simulink library "momentum_dump_lib"  (R2016b)
settings: Solver=VariableStepAuto  StartTime=0.0  StopTime=10.0  RelTol=1e-3
undefined symbols (not defined in the file or in its folder): fsw_params
libraries: vrlib x1, dspmathops x1
settings Model: Creator=unsik  LastModifiedBy=Taylor

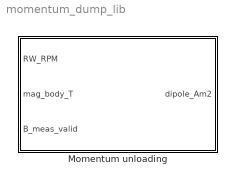
== system momentum_dump_lib ==
  Momentum unloading : Subsystem

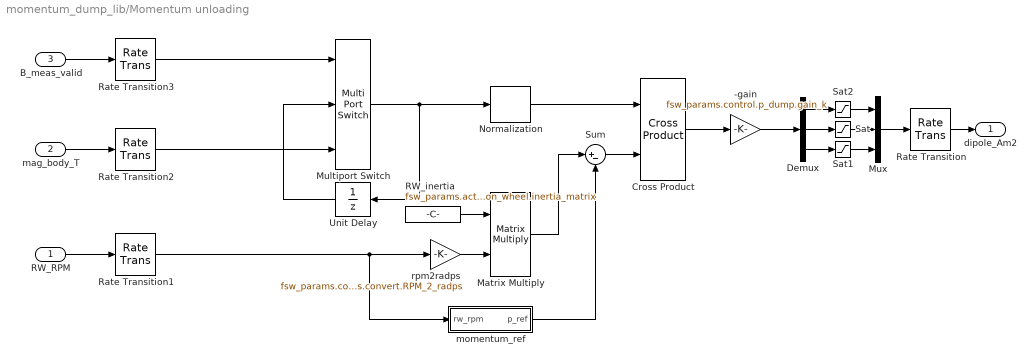
== system momentum_dump_lib/Momentum unloading ==
  RW_RPM : Inport
  mag_body_T : Inport  Port=2
  B_meas_valid : Inport  Port=3
  -gain : Gain  Gain=fsw_params.control.p_dump.gain_k
  Cross Product : vrlib/Utilities/Cross Product
  Demux : Demux  Outputs=3
  Matrix Multiply : Product  Inputs=**  Multiplication=Matrix(*)
  Multiport Switch : MultiPortSwitch  DataPortOrder=Zero-based contiguous  Inputs=2
  Mux : Mux  Inputs=3
  Normalization : dspmathops/Normalization  NormType=Squared 2-norm  Bias=1e-10  NormOver=Each column  Dimension=1  outputDataTypeStr=Inherit: Same as product output  outputLastDataTypeStr=Inherit: Same as product output  outputMin=[]  outputMax=[]  accumDataTypeStr=Inherit: Same as product output  accumLastDataTypeStr=Inherit: Same as product output  roundingMode=Floor  overflowMode=off
  RW_inertia : Constant  Value=fsw_params.actuators.reaction_wheel.inertia_matrix
  Rate Transition : RateTransition  X0=fsw_params.control.p_dump.ic.rt_dipole_Am2
  Rate Transition1 : RateTransition  X0=fsw_params.control.p_dump.ic.rt_rw_RPM  OutPortSampleTime=fsw_params.control.p_dump.sample_time_s
  Rate Transition2 : RateTransition  X0=fsw_params.control.p_dump.ic.rt_mag_body_T  OutPortSampleTime=fsw_params.control.p_dump.sample_time_s
  Rate Transition3 : RateTransition  X0=fsw_params.control.p_dump.ic.rt_B_meas_valid  OutPortSampleTime=fsw_params.control.p_dump.sample_time_s
  Sat : Saturate  UpperLimit=fsw_params.actuators.magnetorquer.max_dipole_y  LowerLimit=-fsw_params.actuators.magnetorquer.max_dipole_y
  Sat1 : Saturate  UpperLimit=fsw_params.actuators.magnetorquer.max_dipole_z  LowerLimit=-fsw_params.actuators.magnetorquer.max_dipole_z
  Sat2 : Saturate  UpperLimit=fsw_params.actuators.magnetorquer.max_dipole_x  LowerLimit=-fsw_params.actuators.magnetorquer.max_dipole_x
  Sum : Sum  Inputs=|+-
  Unit Delay : UnitDelay  InitialCondition=fsw_params.control.p_dump.ic.rt_mag_body_T  SampleTime=-1
  momentum_ref : Subsystem
  rpm2radps : Gain  Gain=fsw_params.constants.convert.RPM_2_radps
  dipole_Am2 : Outport
  wires:
  RW_inertia/1 -> Matrix Multiply/1
  Multiport Switch/1 -> Unit Delay/1, Normalization/1
  rpm2radps/1 -> Matrix Multiply/2
  Sum/1 -> Cross Product/2
  Cross Product/1 -> -gain/1
  Unit Delay/1 -> Multiport Switch/2
  B_meas_valid/1 -> Rate Transition3/1
  mag_body_T/1 -> Rate Transition2/1
  RW_RPM/1 -> Rate Transition1/1
  Rate Transition1/1 -> momentum_ref/1(rw_rpm), rpm2radps/1
  Demux/2 -> Sat/1
  Demux/1 -> Sat2/1
  Demux/3 -> Sat1/1
  Sat1/1 -> Mux/3
  Sat/1 -> Mux/2
  Sat2/1 -> Mux/1
  Mux/1 -> Rate Transition/1
  Rate Transition2/1 -> Multiport Switch/3
  Normalization/1 -> Cross Product/1
  Rate Transition/1 -> dipole_Am2/1
  -gain/1 -> Demux/1
  Matrix Multiply/1 -> Sum/1
  momentum_ref/1(p_ref) -> Sum/2
  Rate Transition3/1 -> Multiport Switch/1

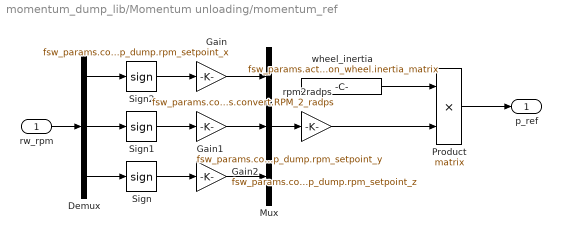
== system momentum_dump_lib/Momentum unloading/momentum_ref ==
  rw_rpm : Inport
  Demux : Demux  Outputs=3
  Gain : Gain  Gain=fsw_params.control.p_dump.rpm_setpoint_x
  Gain1 : Gain  Gain=fsw_params.control.p_dump.rpm_setpoint_y
  Gain2 : Gain  Gain=fsw_params.control.p_dump.rpm_setpoint_z
  Mux : Mux  Inputs=3
  Product : Product  Multiplication=Matrix(*)
  Sign : Signum
  Sign1 : Signum
  Sign2 : Signum
  rpm2radps : Gain  Gain=fsw_params.constants.convert.RPM_2_radps
  wheel_inertia : Constant  Value=fsw_params.actuators.reaction_wheel.inertia_matrix
  p_ref : Outport
  wires:
  rw_rpm/1 -> Demux/1
  Demux/3 -> Sign/1
  Demux/1 -> Sign2/1
  Demux/2 -> Sign1/1
  Sign2/1 -> Gain/1
  Sign/1 -> Gain2/1
  Sign1/1 -> Gain1/1
  Gain2/1 -> Mux/3
  Gain1/1 -> Mux/2
  Gain/1 -> Mux/1
  Mux/1 -> rpm2radps/1
  rpm2radps/1 -> Product/2
  wheel_inertia/1 -> Product/1
  Product/1 -> p_ref/1
